simulink library "lib_transmission2"  (Simulink 4.1.1)
values from neighbouring files (symbols this model uses):
  logFlag = 1    [advSACompMaskInit.m]    (also in advSACompMaskInitR13.m)
undefined symbols (not defined in the file or in its folder): cyc_mph, fc_map_spd, fc_max_trq, fc_spd_scale, fc_trq_scale, fd_inertia, fd_loss, fd_ratio, gb_dnshift_load, gb_dnshift_spd, gb_gear_number_lookup, gb_gears_num, gb_inertia, gb_loss_const, gb_loss_input_spd_coeff, gb_loss_input_trq_coeff, gb_loss_output_spd_coeff, gb_loss_output_trq_coeff, gb_map_spd_out, gb_map_trq_in, gb_map_trq_out, gb_num_init, gb_ratio, gb_shift_delay, gb_spd_scale, gb_trq_scale, gb_upshift_load, gb_upshift_spd, htc_inertia, htc_k_adv, htc_k_adv_coast, htc_lockup, htc_lockup_load, htc_lockup_spd, htc_lu_gear_range, htc_max_coast_tr, htc_min_coast_tr, htc_pump_loss_spd, htc_pump_loss_trq_lockup, htc_pump_loss_trq_unlock, htc_sr, htc_sr_coast, htc_tr, htc_tr_coast, htc_unlock_spd, mc_map_spd, mc_max_trq, mc_overtrq_factor, mc_spd_scale, mc_trq_scale, tc_loss, tc_mc_to_fc_ratio, tx_eff_map, tx_map_spd, tx_map_trq, tx_pg_r, tx_pg_s, tx_speed_dep, vc_clutch_bool, vc_idle_spd ... (+2)
libraries: lib_controls x1, lib_etc x1, lib_controls2 x1, lib_transmission x1
(part 14 of 17)

== system lib_transmission2/gearbox <gb> old/gearbox model & interface/gearbox model/gearing (Nm) (rad/s) ==
  "output shaft torque and speed  (Nm), (rad/s)" : Inport  Port=1  LatchInput=off
  gear ratio : Inport  Port=2  LatchInput=off
  Demux : Demux  Outputs=2  BusSelectionMode=off
  Fcn1 : Fcn  Expr=1/u
  Product2 : Product  Inputs=2  Multiplication=Element-wise(.*)  SaturateOnIntegerOverflow=on
  Product3 : Product  Inputs=2  Multiplication=Element-wise(.*)  SaturateOnIntegerOverflow=on
  input shaft torque (Nm) : Outport  Port=1  InitialOutput=0
  input shaft speed (rad/s) : Outport  Port=2  InitialOutput=0
  wires:
  Product3/1 -> input shaft speed (rad/s)/1
  Product2/1 -> input shaft torque (Nm)/1
  Fcn1/1 -> Product2/2
  "output shaft torque and speed  (Nm), (rad/s)"/1 -> Demux/1
  gear ratio/1 -> Fcn1/1, Product3/2
  Demux/1 -> Product2/1
  Demux/2 -> Product3/1

== system lib_transmission2/gearbox <gb> old/gearbox model & interface/gearbox model/gearing (Nm) (rad/s)1 ==
  input shaft torque (Nm) : Inport  Port=1  LatchInput=off
  input shaft speed (rad/s) : Inport  Port=2  LatchInput=off
  gear ratio : Inport  Port=3  LatchInput=off
  Fcn1 : Fcn  Expr=1/u
  Product2 : Product  Inputs=2  Multiplication=Element-wise(.*)  SaturateOnIntegerOverflow=on
  Product3 : Product  Inputs=2  Multiplication=Element-wise(.*)  SaturateOnIntegerOverflow=on
  output shaft torque (Nm) : Outport  Port=1  InitialOutput=0
  output shaft speed (rad/s) : Outport  Port=2  InitialOutput=0
  wires:
  Fcn1/1 -> Product3/1
  gear ratio/1 -> Product2/2, Fcn1/1
  Product3/1 -> output shaft speed (rad/s)/1
  Product2/1 -> output shaft torque (Nm)/1
  input shaft torque (Nm)/1 -> Product2/1
  input shaft speed (rad/s)/1 -> Product3/2

== system lib_transmission2/gearbox <gb> old/gearbox model & interface/gearbox model/help ==

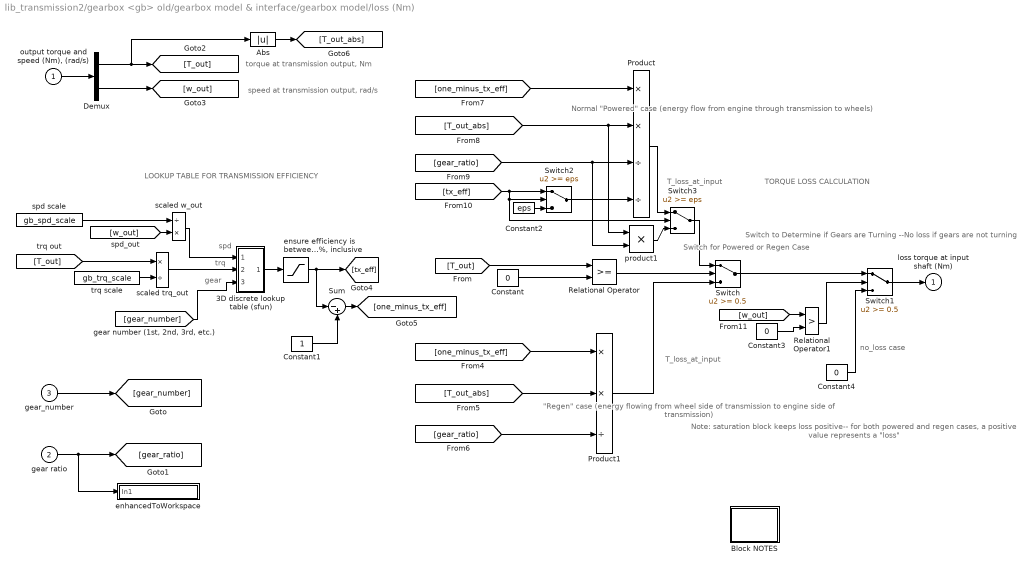
== system lib_transmission2/gearbox <gb> old/gearbox model & interface/gearbox model/loss (Nm) ==
  note: TORQUE LOSS CALCULATION
  note: gear
  note: trq
  note: spd
  note: torque at transmission output, Nm
  note: speed at transmission output, rad/s
  note: no_loss case
  note: Note: saturation block keeps
      | loss positive-- for both powered
      | and regen cases, a
      | positive value represents a "loss"
  note: Switch for Powered
      |  or Regen Case
  note: Switch to Determine
      | if Gears are Turning
      | --No loss if gears
      | are not turning
  note: Normal "Powered" case
      | (energy flow from engine
      | through transmission to wheels)
  note: T_loss_at_input
  note: "Regen" case
      | (energy flowing from
      | wheel side of transmission
      | to engine side of transmission)
  note: T_loss_at_input
  note: LOOKUP TABLE FOR TRANSMISSION EFFICIENCY
  "output torque and speed (Nm), (rad/s)" : Inport  Port=1  LatchInput=off
  gear ratio : Inport  Port=2  LatchInput=off
  gear_number : Inport  Port=3  LatchInput=off
  3D discrete lookup table (sfun) : Subsystem  mask{tx_map_spd=tx_map_spd, tx_map_trq=tx_map_trq, tx_eff_map=tx_eff_map}
      mask prompts: tx_map_spd "Row Lookup"; tx_map_trq "Column Lookup"; tx_eff_map "Lookup Matrix"
      settings: RTWFcnNameOpts=Auto  RTWFileNameOpts=Auto
  Abs : Abs  SaturateOnIntegerOverflow=on
  Block NOTES : Subsystem
      settings: RTWFcnNameOpts=Auto  RTWFileNameOpts=Auto
      mask Display: disp('Block\nNOTES')
  Constant : Constant  Value=0
  Constant1 : Constant  Value=1
  Constant2 : Constant  Value=eps
  Constant3 : Constant  Value=0
  Constant4 : Constant  Value=0
  Demux : Demux  Outputs=2  BusSelectionMode=off
  Product : Product  Inputs=**//  Multiplication=Element-wise(.*)  SaturateOnIntegerOverflow=on
  Product1 : Product  Inputs=**/  Multiplication=Element-wise(.*)  SaturateOnIntegerOverflow=on
  Relational Operator : RelationalOperator  Operator=>=
  Relational Operator1 : RelationalOperator  Operator=>
  Sum : Sum  Inputs=|-+  SaturateOnIntegerOverflow=on
  Switch : Switch  Threshold=0.5
  Switch1 : Switch  Threshold=0.5
  Switch2 : Switch  Threshold=eps
  Switch3 : Switch  Threshold=eps
  enhancedToWorkspace : Subsystem  TreatAsAtomicUnit=on  mask(enhancedToWorkspace){generalName=generalName, specificName=current_gear_ratio, logFlag=logFlag}
      mask prompts: generalName "General Name [char-evaluated]"; specificName "Specific Name [char-literal]"; logFlag "Enable flag (1=on,0=off)"
      mask help: A wrapper for the Simulink "To Workspace" block that allows you to evaluate the name of the variable to log to workspace. This is useful to avoid the double logging errors that occur when you pull in two library models that attempt to log to the same variable.
      mask init:
      | enhancedToWsMaker
      settings: CopyFcn=breakLinkCopyFcn  ParentCloseFcn=breakLinkParCloseFcn  RTWFcnNameOpts=Auto  RTWFileNameOpts=Auto
      mask Help:
      | <h2>Enhanced To Workspace Block</h2>
      | <h3>Parameters</h3>
      | <UL>
      | <li><b>General Name:</b> This is the more general name of the variable. Variables are saved to the workspace as <i>generalName_specificName</i>. Note that this is an evaluated variable. If you would like to type in the value directly, it must be surrounded with single quotes. Otherwise you can input the name of a variable containing a char string.</li>
      | <li><b>Specific Name:</b> This is the specific name of the variable. Note that this is input as a char literal (i.e., you don't need quotes).</li>
      | <li><b>Enable Flag:</b> This flag should have the value of 0 or 1. If 0, the variable will not be logged to the workspace. If 1, the variable will be logged. This is done so that variable logging can be turned off to improve speed.</li>
      | </ul>
      | <h3>Overview</h3>
      | <p>The enhanced to workspace block was put together to allow one to dynamically resolve variable names at run time in simulink. This is most powerful when used in conjunction with a masked subsystem to allow multiple instances of that masked subsytem to be used in the same model. The strategy is to set the generalName in the block mask which will allow the block to change the general name for all variable logging on the fly.
      | <h3>Helper Files</h3>
      | <p>Three m-files are required by the enhancedToWorkspace block. These files are located in the &lt; ADVISOR root &gt;/GUI directory :
      | <ul>
      | <li><i>enhancedToWsMaker.m</i> This file runs the mask initialization for the block</li>
      | <li><i>breakLinkCopyFcn.m</i> This file is used by the block callback when the simulink block is copied. It is necessary to break the link to the enhancedToWorkspace similar to the To Workspace block in order for it to be able to configure itself. (Try copying simulink's To Workspace block--it is impossible to make a link)</li>
      | <li><i>breakLinkParCloseFcn.m</i> This file is similar to the breakLinkCopyFcn and is used when a parent system is closed</li>
      | </ul>
      | <hr>
      | 
      | <p>Created 2003-Jan-21, Michael Patrick O'Keefe, NREL</p>
      | 
      | <!--
      | <VARDEF>
      | <H3>var_name</H3>
      | <UL>
      | <LI><B>data type</B> data type here</LI>
      | <LI><B>units</B> units here</LI>
      | <LI><B>vehicle type</B> vehicle type here</LI>
      | <LI><B>description</B> description here</LI>
      | </UL>
      | </VARDEF>
      | -->
      mask Display: disp([generalName,'_',specificName])
  "ensure efficiency is between  0% and 100%, inclusive" : Saturate  UpperLimit=1  LowerLimit=0  LinearizeAsGain=on
  product1 : Product  Inputs=2  Multiplication=Element-wise(.*)  SaturateOnIntegerOverflow=on
  scaled trq_out : Product  Inputs=*/  Multiplication=Element-wise(.*)  SaturateOnIntegerOverflow=on
  scaled w_out : Product  Inputs=/*  Multiplication=Element-wise(.*)  SaturateOnIntegerOverflow=on
  spd scale : Constant  Value=gb_spd_scale
  trq scale : Constant  Value=gb_trq_scale
  loss torque at input shaft (Nm) : Outport  Port=1  InitialOutput=0
  wires:
  product1/1 -> Switch3/3
  Product/1 -> Switch3/1
  Switch3/1 -> Switch/1
  Constant2/1 -> Switch2/3
  [tx_eff] -> Switch3/2, Switch2/2, Switch2/1
  Switch2/1 -> Product/4
  gear_number/1 -> [gear_number]
  gear ratio/1 -> [gear_ratio], enhancedToWorkspace/1(In1)
  spd scale/1 -> scaled w_out/1
  [w_out] -> scaled w_out/2
  Sum/1 -> [one_minus_tx_eff]
  Constant1/1 -> Sum/2
  trq scale/1 -> scaled trq_out/2
  scaled trq_out/1 -> 3D discrete lookup table (sfun)/2(lookup trq (Nm))
  [T_out] -> scaled trq_out/1
  scaled w_out/1 -> 3D discrete lookup table (sfun)/1(lookup speed (rad/s))
  "ensure efficiency is between  0% and 100%, inclusive"/1 -> Sum/1, [tx_eff]
  3D discrete lookup table (sfun)/1(tx_eff) -> "ensure efficiency is between  0% and 100%, inclusive"/1
  Switch/1 -> Switch1/1
  Abs/1 -> [T_out_abs]
  Demux/1 -> Abs/1, [T_out]
  Relational Operator1/1 -> Switch1/2
  Constant3/1 -> Relational Operator1/2
  [w_out] -> Relational Operator1/1
  Constant4/1 -> Switch1/3
  Switch1/1 -> loss torque at input shaft (Nm)/1
  [gear_ratio] -> product1/2, Product/3
  [T_out_abs] -> product1/1, Product/2
  [one_minus_tx_eff] -> Product/1
  [T_out_abs] -> Product1/2
  [gear_ratio] -> Product1/3
  [one_minus_tx_eff] -> Product1/1
  Product1/1 -> Switch/3
  [T_out] -> Relational Operator/1
  Constant/1 -> Relational Operator/2
  Relational Operator/1 -> Switch/2
  [gear_number] -> 3D discrete lookup table (sfun)/3("gear_number  (e.g., 1, 2, 3)")
  Demux/2 -> [w_out]
  "output torque and speed (Nm), (rad/s)"/1 -> Demux/1

== system lib_transmission2/hydraulic torque converter <htc>/conventional HTC  and Interface/htc model/SR ==
  T,w req out : Inport  Port=1  LatchInput=off
  w in : Inport  Port=2  LatchInput=off
  >0 : Saturate  UpperLimit=inf  LowerLimit=eps  LinearizeAsGain=on
  Constant : Constant  Orientation=left  Value=0
  Constant1 : Constant  Value=vc_idle_spd+eps
  Constant3 : Constant  Value=1
  K_adv : Subsystem
      settings: RTWFcnNameOpts=Auto  RTWFileNameOpts=Auto
  K_adv_coast : Subsystem
      settings: RTWFcnNameOpts=Auto  RTWFileNameOpts=Auto
  Logical Operator : Logic  Operator=NOT  Inputs=1
  Logical Operator1 : Logic  Operator=NOT  Inputs=1
  MinMax : MinMax  Function=min  Inputs=2
  Relational Operator : RelationalOperator  Operator=>=
  SR Look-Up Table SR=wout/win : Lookup  InputValues=htc_k_adv  OutputValues=htc_sr
  SR Look-Up Table SR=wout/win coast : Lookup  InputValues=fliplr(htc_k_adv_coast)  OutputValues=fliplr(htc_sr_coast)
  SRmax= wout/win,min : Product  Inputs=*/  Multiplication=Element-wise(.*)  SaturateOnIntegerOverflow=on
  T : Selector  InputType=Vector  ElementSrc=Internal  Elements=1  RowSrc=Internal  Rows=1  ColumnSrc=Internal  Columns=1  InputPortWidth=2
  enhancedToWorkspace1 : Subsystem  TreatAsAtomicUnit=on  mask(enhancedToWorkspace){generalName=generalName, specificName=coasting, logFlag=logFlag}
      mask prompts: generalName "General Name [char-evaluated]"; specificName "Specific Name [char-literal]"; logFlag "Enable flag (1=on,0=off)"
      mask help: A wrapper for the Simulink "To Workspace" block that allows you to evaluate the name of the variable to log to workspace. This is useful to avoid the double logging errors that occur when you pull in two library models that attempt to log to the same variable.
      mask init:
      | enhancedToWsMaker
      settings: CopyFcn=breakLinkCopyFcn  ParentCloseFcn=breakLinkParCloseFcn  RTWFcnNameOpts=Auto  RTWFileNameOpts=Auto
      mask Help:
      | <h2>Enhanced To Workspace Block</h2>
      | <h3>Parameters</h3>
      | <UL>
      | <li><b>General Name:</b> This is the more general name of the variable. Variables are saved to the workspace as <i>generalName_specificName</i>. Note that this is an evaluated variable. If you would like to type in the value directly, it must be surrounded with single quotes. Otherwise you can input the name of a variable containing a char string.</li>
      | <li><b>Specific Name:</b> This is the specific name of the variable. Note that this is input as a char literal (i.e., you don't need quotes).</li>
      | <li><b>Enable Flag:</b> This flag should have the value of 0 or 1. If 0, the variable will not be logged to the workspace. If 1, the variable will be logged. This is done so that variable logging can be turned off to improve speed.</li>
      | </ul>
      | <h3>Overview</h3>
      | <p>The enhanced to workspace block was put together to allow one to dynamically resolve variable names at run time in simulink. This is most powerful when used in conjunction with a masked subsystem to allow multiple instances of that masked subsytem to be used in the same model. The strategy is to set the generalName in the block mask which will allow the block to change the general name for all variable logging on the fly.
      | <h3>Helper Files</h3>
      | <p>Three m-files are required by the enhancedToWorkspace block. These files are located in the &lt; ADVISOR root &gt;/GUI directory :
      | <ul>
      | <li><i>enhancedToWsMaker.m</i> This file runs the mask initialization for the block</li>
      | <li><i>breakLinkCopyFcn.m</i> This file is used by the block callback when the simulink block is copied. It is necessary to break the link to the enhancedToWorkspace similar to the To Workspace block in order for it to be able to configure itself. (Try copying simulink's To Workspace block--it is impossible to make a link)</li>
      | <li><i>breakLinkParCloseFcn.m</i> This file is similar to the breakLinkCopyFcn and is used when a parent system is closed</li>
      | </ul>
      | <hr>
      | 
      | <p>Created 2003-Jan-21, Michael Patrick O'Keefe, NREL</p>
      | 
      | <!--
      | <VARDEF>
      | <H3>var_name</H3>
      | <UL>
      | <LI><B>data type</B> data type here</LI>
      | <LI><B>units</B> units here</LI>
      | <LI><B>vehicle type</B> vehicle type here</LI>
      | <LI><B>description</B> description here</LI>
      | </UL>
      | </VARDEF>
      | -->
      mask Display: disp([generalName,'_',specificName])
  enhancedToWorkspace2 : Subsystem  TreatAsAtomicUnit=on  mask(enhancedToWorkspace){generalName=generalName, specificName=locked, logFlag=logFlag}
      mask prompts: generalName "General Name [char-evaluated]"; specificName "Specific Name [char-literal]"; logFlag "Enable flag (1=on,0=off)"
      mask help: A wrapper for the Simulink "To Workspace" block that allows you to evaluate the name of the variable to log to workspace. This is useful to avoid the double logging errors that occur when you pull in two library models that attempt to log to the same variable.
      mask init:
      | enhancedToWsMaker
      settings: CopyFcn=breakLinkCopyFcn  ParentCloseFcn=breakLinkParCloseFcn  RTWFcnNameOpts=Auto  RTWFileNameOpts=Auto
      mask Help:
      | <h2>Enhanced To Workspace Block</h2>
      | <h3>Parameters</h3>
      | <UL>
      | <li><b>General Name:</b> This is the more general name of the variable. Variables are saved to the workspace as <i>generalName_specificName</i>. Note that this is an evaluated variable. If you would like to type in the value directly, it must be surrounded with single quotes. Otherwise you can input the name of a variable containing a char string.</li>
      | <li><b>Specific Name:</b> This is the specific name of the variable. Note that this is input as a char literal (i.e., you don't need quotes).</li>
      | <li><b>Enable Flag:</b> This flag should have the value of 0 or 1. If 0, the variable will not be logged to the workspace. If 1, the variable will be logged. This is done so that variable logging can be turned off to improve speed.</li>
      | </ul>
      | <h3>Overview</h3>
      | <p>The enhanced to workspace block was put together to allow one to dynamically resolve variable names at run time in simulink. This is most powerful when used in conjunction with a masked subsystem to allow multiple instances of that masked subsytem to be used in the same model. The strategy is to set the generalName in the block mask which will allow the block to change the general name for all variable logging on the fly.
      | <h3>Helper Files</h3>
      | <p>Three m-files are required by the enhancedToWorkspace block. These files are located in the &lt; ADVISOR root &gt;/GUI directory :
      | <ul>
      | <li><i>enhancedToWsMaker.m</i> This file runs the mask initialization for the block</li>
      | <li><i>breakLinkCopyFcn.m</i> This file is used by the block callback when the simulink block is copied. It is necessary to break the link to the enhancedToWorkspace similar to the To Workspace block in order for it to be able to configure itself. (Try copying simulink's To Workspace block--it is impossible to make a link)</li>
      | <li><i>breakLinkParCloseFcn.m</i> This file is similar to the breakLinkCopyFcn and is used when a parent system is closed</li>
      | </ul>
      | <hr>
      | 
      | <p>Created 2003-Jan-21, Michael Patrick O'Keefe, NREL</p>
      | 
      | <!--
      | <VARDEF>
      | <H3>var_name</H3>
      | <UL>
      | <LI><B>data type</B> data type here</LI>
      | <LI><B>units</B> units here</LI>
      | <LI><B>vehicle type</B> vehicle type here</LI>
      | <LI><B>description</B> description here</LI>
      | </UL>
      | </VARDEF>
      | -->
      mask Display: disp([generalName,'_',specificName])
  if coasting : Switch  Threshold=eps
  "locked up, then SR=1" : Switch  Threshold=eps
  min,max : Saturate  UpperLimit=inf  LowerLimit=1  LinearizeAsGain=on
  shifting SR : Subsystem
      settings: RTWFcnNameOpts=Auto  RTWFileNameOpts=Auto
  wout,req : Selector  InputType=Vector  ElementSrc=Internal  Elements=2  RowSrc=Internal  Rows=1  ColumnSrc=Internal  Columns=1  InputPortWidth=2
  SR : Outport  Port=1  InitialOutput=0
  coasting : Outport  Port=2  InitialOutput=0
  wires:
  K_adv/1(K_adv) -> SR Look-Up Table SR=wout/win/1
  Logical Operator1/1 -> coasting/1, enhancedToWorkspace1/1(In1)
  >0/1 -> SR/1
  if coasting/1 -> >0/1
  K_adv_coast/1(K_adv_coast) -> SR Look-Up Table SR=wout/win coast/1
  MinMax/1 -> if coasting/3
  min,max/1 -> MinMax/1
  wout,req/1 -> SRmax= wout/win,min/1
  Constant1/1 -> SRmax= wout/win,min/2
  SRmax= wout/win,min/1 -> MinMax/2
  shifting SR/1(SR limited) -> if coasting/1
  "locked up, then SR=1"/1 -> shifting SR/3(SR)
  w in/1 -> shifting SR/2(w in)
  SR Look-Up Table SR=wout/win/1 -> "locked up, then SR=1"/1
  Constant3/1 -> "locked up, then SR=1"/3
  Logical Operator/1 -> "locked up, then SR=1"/2
  Relational Operator/1 -> Logical Operator1/1, if coasting/2
  T/1 -> Relational Operator/1
  Constant/1 -> Relational Operator/2
  SR Look-Up Table SR=wout/win coast/1 -> min,max/1
  T,w req out/1 -> shifting SR/1(T,w req out), K_adv/1("Req'd output trq and spd (Nm), (rad/s)"), wout,req/1, K_adv_coast/1("Req'd output trq and spd (Nm), (rad/s)"), T/1
  [locked_up] -> Logical Operator/1, enhancedToWorkspace2/1(In1)

== system lib_transmission2/hydraulic torque converter <htc>/conventional HTC  and Interface/htc model/T, shifting ==
  TR : Inport  Port=1  LatchInput=off
  Req'd  input trq : Inport  Port=2  LatchInput=off
  Req'd output trq : Inport  Port=3  LatchInput=off
  htc_spd_in_a : Inport  Port=4  LatchInput=off
  SR : Inport  Port=5  LatchInput=off
  Memory : Memory  X0=0  InheritSampleTime=off
      settings: RTWStateStorageClass=Auto
  Memory1 : Memory  X0=0  InheritSampleTime=off
      settings: RTWStateStorageClass=Auto
  MinMax : MinMax  Function=min  Inputs=2
  TR Look-Up Table TR=Tout/Tin : Lookup  InputValues=htc_sr  OutputValues=htc_tr
  T_max : Subsystem
      settings: RTWFcnNameOpts=Auto  RTWFileNameOpts=Auto
  Tin*TR= Tout,req : Product  Inputs=2  Multiplication=Element-wise(.*)  SaturateOnIntegerOverflow=on
  engine speed estimator : Subsystem
      settings: RTWFcnNameOpts=Auto  RTWFileNameOpts=Auto
  "shifting, override zero Trequest" : Switch  Threshold=eps
  T req : Outport  Port=1
  wires:
  Tin*TR= Tout,req/1 -> Memory/1
  TR/1 -> Tin*TR= Tout,req/2
  Req'd  input trq/1 -> Tin*TR= Tout,req/1
  Memory/1 -> "shifting, override zero Trequest"/1
  T_max/1(T_max max gain from htc) -> MinMax/2
  "shifting, override zero Trequest"/1 -> MinMax/1
  TR Look-Up Table TR=Tout/Tin/1 -> T_max/2(TR)
  MinMax/1 -> T req/1
  engine speed estimator/1(Out1) -> T_max/1(w_APU)
  Memory1/1 -> TR Look-Up Table TR=Tout/Tin/1
  SR/1 -> Memory1/1
  htc_spd_in_a/1 -> engine speed estimator/1(htc_spd_in_a)
  Req'd output trq/1 -> "shifting, override zero Trequest"/3
  [shifting] -> "shifting, override zero Trequest"/2

== system lib_transmission2/hydraulic torque converter <htc>/conventional HTC  and Interface/htc model/TR ==
  SR : Inport  Port=1  LatchInput=off
  coasting : Inport  Port=2  LatchInput=off
  1/SR*TR  for coast : Fcn  Expr=1/u
  Constant3 : Constant  Value=1
  Logical Operator : Logic  Operator=NOT  Inputs=1
  Logical Operator1 : Logic  Operator=NOT  Inputs=1
  TR Look-Up Table TR=Tout/Tin : Lookup  InputValues=htc_sr  OutputValues=htc_tr
  TR Look-Up Table TR=Tout/Tin coast : Lookup  InputValues=htc_sr_coast  OutputValues=htc_tr_coast
  effic=SR*TR : Product  Inputs=**  Multiplication=Element-wise(.*)  SaturateOnIntegerOverflow=on
  enhancedToWorkspace2 : Subsystem  TreatAsAtomicUnit=on  mask(enhancedToWorkspace){generalName=generalName, specificName=efficiency, logFlag=logFlag}
      mask prompts: generalName "General Name [char-evaluated]"; specificName "Specific Name [char-literal]"; logFlag "Enable flag (1=on,0=off)"
      mask help: A wrapper for the Simulink "To Workspace" block that allows you to evaluate the name of the variable to log to workspace. This is useful to avoid the double logging errors that occur when you pull in two library models that attempt to log to the same variable.
      mask init:
      | enhancedToWsMaker
      settings: CopyFcn=breakLinkCopyFcn  ParentCloseFcn=breakLinkParCloseFcn  RTWFcnNameOpts=Auto  RTWFileNameOpts=Auto
      mask Help:
      | <h2>Enhanced To Workspace Block</h2>
      | <h3>Parameters</h3>
      | <UL>
      | <li><b>General Name:</b> This is the more general name of the variable. Variables are saved to the workspace as <i>generalName_specificName</i>. Note that this is an evaluated variable. If you would like to type in the value directly, it must be surrounded with single quotes. Otherwise you can input the name of a variable containing a char string.</li>
      | <li><b>Specific Name:</b> This is the specific name of the variable. Note that this is input as a char literal (i.e., you don't need quotes).</li>
      | <li><b>Enable Flag:</b> This flag should have the value of 0 or 1. If 0, the variable will not be logged to the workspace. If 1, the variable will be logged. This is done so that variable logging can be turned off to improve speed.</li>
      | </ul>
      | <h3>Overview</h3>
      | <p>The enhanced to workspace block was put together to allow one to dynamically resolve variable names at run time in simulink. This is most powerful when used in conjunction with a masked subsystem to allow multiple instances of that masked subsytem to be used in the same model. The strategy is to set the generalName in the block mask which will allow the block to change the general name for all variable logging on the fly.
      | <h3>Helper Files</h3>
      | <p>Three m-files are required by the enhancedToWorkspace block. These files are located in the &lt; ADVISOR root &gt;/GUI directory :
      | <ul>
      | <li><i>enhancedToWsMaker.m</i> This file runs the mask initialization for the block</li>
      | <li><i>breakLinkCopyFcn.m</i> This file is used by the block callback when the simulink block is copied. It is necessary to break the link to the enhancedToWorkspace similar to the To Workspace block in order for it to be able to configure itself. (Try copying simulink's To Workspace block--it is impossible to make a link)</li>
      | <li><i>breakLinkParCloseFcn.m</i> This file is similar to the breakLinkCopyFcn and is used when a parent system is closed</li>
      | </ul>
      | <hr>
      | 
      | <p>Created 2003-Jan-21, Michael Patrick O'Keefe, NREL</p>
      | 
      | <!--
      | <VARDEF>
      | <H3>var_name</H3>
      | <UL>
      | <LI><B>data type</B> data type here</LI>
      | <LI><B>units</B> units here</LI>
      | <LI><B>vehicle type</B> vehicle type here</LI>
      | <LI><B>description</B> description here</LI>
      | </UL>
      | </VARDEF>
      | -->
      mask Display: disp([generalName,'_',specificName])
  if coasting : Switch  Threshold=eps
  if coasting1 : Switch  Threshold=eps
  "locked up, then TR=1" : Switch  Threshold=eps
  min,max : Saturate  UpperLimit=htc_max_coast_tr  LowerLimit=htc_min_coast_tr  LinearizeAsGain=on
  TR : Outport  Port=1  InitialOutput=0
  tag scope: htc_efficiency=scoped
  wires:
  if coasting1/1 -> [htc_efficiency], enhancedToWorkspace2/1(In1)
  1/SR*TR  for coast/1 -> if coasting1/3
  effic=SR*TR/1 -> 1/SR*TR  for coast/1, if coasting1/1
  Logical Operator1/1 -> if coasting1/2, if coasting/2
  if coasting/1 -> effic=SR*TR/2, TR/1
  coasting/1 -> Logical Operator1/1
  SR/1 -> effic=SR*TR/1, TR Look-Up Table TR=Tout/Tin/1, TR Look-Up Table TR=Tout/Tin coast/1
  min,max/1 -> if coasting/3
  TR Look-Up Table TR=Tout/Tin coast/1 -> min,max/1
  "locked up, then TR=1"/1 -> if coasting/1
  Logical Operator/1 -> "locked up, then TR=1"/2
  [locked_up] -> Logical Operator/1
  Constant3/1 -> "locked up, then TR=1"/3
  TR Look-Up Table TR=Tout/Tin/1 -> "locked up, then TR=1"/1

== system lib_transmission2/hydraulic torque converter <htc>/conventional HTC  and Interface/htc model/effect of inertia (Nm) ==
  note: This block computes the torque required to overcome the inertia of the
      | turbine (plus 1/2 fluid in htc).
  turbine/output speed (rad/s) : Inport  Port=1  LatchInput=off
  Constant : Constant  Value=htc_inertia
  Product : Product  Inputs=2  Multiplication=Element-wise(.*)  SaturateOnIntegerOverflow=on
  d/dt : Derivative
  inertia torque (Nm) : Outport  Port=1  InitialOutput=0
  wires:
  Product/1 -> inertia torque (Nm)/1
  Constant/1 -> Product/2
  turbine/output speed (rad/s)/1 -> d/dt/1
  d/dt/1 -> Product/1

== system lib_transmission2/hydraulic torque converter <htc>/conventional HTC  and Interface/htc model/enhancedToWorkspace ==
  In1 : Inport  Port=1  LatchInput=off
  To Workspace : ToWorkspace  VariableName=htc_trq_in_a  SampleTime=-1  SaveFormat=Array
  wires:
  In1/1 -> To Workspace/1

== system lib_transmission2/hydraulic torque converter <htc>/conventional HTC  and Interface/htc model/enhancedToWorkspace1 ==
  In1 : Inport  Port=1  LatchInput=off
  To Workspace : ToWorkspace  VariableName=htc_spd_in_a  SampleTime=-1  SaveFormat=Array
  wires:
  In1/1 -> To Workspace/1

== system lib_transmission2/hydraulic torque converter <htc>/conventional HTC  and Interface/htc model/enhancedToWorkspace10 ==
  In1 : Inport  Port=1  LatchInput=off
  To Workspace : ToWorkspace  VariableName=htc_spd_out_a  SampleTime=-1  SaveFormat=Array
  wires:
  In1/1 -> To Workspace/1

== system lib_transmission2/hydraulic torque converter <htc>/conventional HTC  and Interface/htc model/enhancedToWorkspace2 ==
  In1 : Inport  Port=1  LatchInput=off
  To Workspace : ToWorkspace  VariableName=htc_trq_out_r  SampleTime=-1  SaveFormat=Array
  wires:
  In1/1 -> To Workspace/1

== system lib_transmission2/hydraulic torque converter <htc>/conventional HTC  and Interface/htc model/enhancedToWorkspace3 ==
  In1 : Inport  Port=1  LatchInput=off
  To Workspace : ToWorkspace  VariableName=htc_spd_out_r  SampleTime=-1  SaveFormat=Array
  wires:
  In1/1 -> To Workspace/1

== system lib_transmission2/hydraulic torque converter <htc>/conventional HTC  and Interface/htc model/enhancedToWorkspace4 ==
  In1 : Inport  Port=1  LatchInput=off
  To Workspace : ToWorkspace  VariableName=htc_sr_hist  SampleTime=-1  SaveFormat=Array
  wires:
  In1/1 -> To Workspace/1

== system lib_transmission2/hydraulic torque converter <htc>/conventional HTC  and Interface/htc model/enhancedToWorkspace5 ==
  In1 : Inport  Port=1  LatchInput=off
  To Workspace : ToWorkspace  VariableName=htc_tr_hist  SampleTime=-1  SaveFormat=Array
  wires:
  In1/1 -> To Workspace/1

== system lib_transmission2/hydraulic torque converter <htc>/conventional HTC  and Interface/htc model/enhancedToWorkspace6 ==
  In1 : Inport  Port=1  LatchInput=off
  To Workspace : ToWorkspace  VariableName=htc_spd_in_r  SampleTime=-1  SaveFormat=Array
  wires:
  In1/1 -> To Workspace/1

== system lib_transmission2/hydraulic torque converter <htc>/conventional HTC  and Interface/htc model/enhancedToWorkspace7 ==
  In1 : Inport  Port=1  LatchInput=off
  To Workspace : ToWorkspace  VariableName=htc_trq_in_r  SampleTime=-1  SaveFormat=Array
  wires:
  In1/1 -> To Workspace/1

== system lib_transmission2/hydraulic torque converter <htc>/conventional HTC  and Interface/htc model/enhancedToWorkspace8 ==
  In1 : Inport  Port=1  LatchInput=off
  To Workspace : ToWorkspace  VariableName=htc_trq_inertia  SampleTime=-1  SaveFormat=Array
  wires:
  In1/1 -> To Workspace/1

== system lib_transmission2/hydraulic torque converter <htc>/conventional HTC  and Interface/htc model/enhancedToWorkspace9 ==
  In1 : Inport  Port=1  LatchInput=off
  To Workspace : ToWorkspace  VariableName=htc_trq_out_a  SampleTime=-1  SaveFormat=Array
  wires:
  In1/1 -> To Workspace/1

== system lib_transmission2/hydraulic torque converter <htc> HEV/HTC for parallel HEV and Interface/model for parallel HEV/Block NOTES ==
  note: This block predicts the relative speed of the HTC input (pump) and output
      | (turbine).  Torque converter lockup is modeled.

== system lib_transmission2/hydraulic torque converter <htc> HEV/HTC for parallel HEV and Interface/model for parallel HEV/SR ==
  T,w req out : Inport  Port=1  LatchInput=off
  w in : Inport  Port=2  LatchInput=off
  >0 : Saturate  UpperLimit=inf  LowerLimit=eps  LinearizeAsGain=on
  Constant : Constant  Orientation=left  Value=0
  Constant1 : Constant  Value=vc_idle_spd+eps
  Constant3 : Constant  Value=1
  K_adv : Subsystem
      settings: RTWFcnNameOpts=Auto  RTWFileNameOpts=Auto
  K_adv_coast : Subsystem
      settings: RTWFcnNameOpts=Auto  RTWFileNameOpts=Auto
  Logical Operator : Logic  Operator=NOT  Inputs=1
  Logical Operator1 : Logic  Operator=NOT  Inputs=1
  MinMax : MinMax  Function=min  Inputs=2
  Relational Operator : RelationalOperator  Operator=>=
  SR Look-Up Table SR=wout/win : Lookup  InputValues=htc_k_adv  OutputValues=htc_sr
  SR Look-Up Table SR=wout/win coast : Lookup  InputValues=fliplr(htc_k_adv_coast)  OutputValues=fliplr(htc_sr_coast)
  SRmax= wout/win,min : Product  Inputs=*/  Multiplication=Element-wise(.*)  SaturateOnIntegerOverflow=on
  T : Selector  InputType=Vector  ElementSrc=Internal  Elements=1  RowSrc=Internal  Rows=1  ColumnSrc=Internal  Columns=1  InputPortWidth=2
  enhancedToWorkspace : Subsystem  TreatAsAtomicUnit=on  mask(enhancedToWorkspace){generalName=generalName, specificName=locked, logFlag=logFlag}
      mask prompts: generalName "General Name [char-evaluated]"; specificName "Specific Name [char-literal]"; logFlag "Enable flag (1=on,0=off)"
      mask help: A wrapper for the Simulink "To Workspace" block that allows you to evaluate the name of the variable to log to workspace. This is useful to avoid the double logging errors that occur when you pull in two library models that attempt to log to the same variable.
      mask init:
      | enhancedToWsMaker
      settings: CopyFcn=breakLinkCopyFcn  ParentCloseFcn=breakLinkParCloseFcn  RTWFcnNameOpts=Auto  RTWFileNameOpts=Auto
      mask Help:
      | <h2>Enhanced To Workspace Block</h2>
      | <h3>Parameters</h3>
      | <UL>
      | <li><b>General Name:</b> This is the more general name of the variable. Variables are saved to the workspace as <i>generalName_specificName</i>. Note that this is an evaluated variable. If you would like to type in the value directly, it must be surrounded with single quotes. Otherwise you can input the name of a variable containing a char string.</li>
      | <li><b>Specific Name:</b> This is the specific name of the variable. Note that this is input as a char literal (i.e., you don't need quotes).</li>
      | <li><b>Enable Flag:</b> This flag should have the value of 0 or 1. If 0, the variable will not be logged to the workspace. If 1, the variable will be logged. This is done so that variable logging can be turned off to improve speed.</li>
      | </ul>
      | <h3>Overview</h3>
      | <p>The enhanced to workspace block was put together to allow one to dynamically resolve variable names at run time in simulink. This is most powerful when used in conjunction with a masked subsystem to allow multiple instances of that masked subsytem to be used in the same model. The strategy is to set the generalName in the block mask which will allow the block to change the general name for all variable logging on the fly.
      | <h3>Helper Files</h3>
      | <p>Three m-files are required by the enhancedToWorkspace block. These files are located in the &lt; ADVISOR root &gt;/GUI directory :
      | <ul>
      | <li><i>enhancedToWsMaker.m</i> This file runs the mask initialization for the block</li>
      | <li><i>breakLinkCopyFcn.m</i> This file is used by the block callback when the simulink block is copied. It is necessary to break the link to the enhancedToWorkspace similar to the To Workspace block in order for it to be able to configure itself. (Try copying simulink's To Workspace block--it is impossible to make a link)</li>
      | <li><i>breakLinkParCloseFcn.m</i> This file is similar to the breakLinkCopyFcn and is used when a parent system is closed</li>
      | </ul>
      | <hr>
      | 
      | <p>Created 2003-Jan-21, Michael Patrick O'Keefe, NREL</p>
      | 
      | <!--
      | <VARDEF>
      | <H3>var_name</H3>
      | <UL>
      | <LI><B>data type</B> data type here</LI>
      | <LI><B>units</B> units here</LI>
      | <LI><B>vehicle type</B> vehicle type here</LI>
      | <LI><B>description</B> description here</LI>
      | </UL>
      | </VARDEF>
      | -->
      mask Display: disp([generalName,'_',specificName])
  enhancedToWorkspace1 : Subsystem  TreatAsAtomicUnit=on  mask(enhancedToWorkspace){generalName=generalName, specificName=coasting, logFlag=logFlag}
      mask prompts: generalName "General Name [char-evaluated]"; specificName "Specific Name [char-literal]"; logFlag "Enable flag (1=on,0=off)"
      mask help: A wrapper for the Simulink "To Workspace" block that allows you to evaluate the name of the variable to log to workspace. This is useful to avoid the double logging errors that occur when you pull in two library models that attempt to log to the same variable.
      mask init:
      | enhancedToWsMaker
      settings: CopyFcn=breakLinkCopyFcn  ParentCloseFcn=breakLinkParCloseFcn  RTWFcnNameOpts=Auto  RTWFileNameOpts=Auto
      mask Help:
      | <h2>Enhanced To Workspace Block</h2>
      | <h3>Parameters</h3>
      | <UL>
      | <li><b>General Name:</b> This is the more general name of the variable. Variables are saved to the workspace as <i>generalName_specificName</i>. Note that this is an evaluated variable. If you would like to type in the value directly, it must be surrounded with single quotes. Otherwise you can input the name of a variable containing a char string.</li>
      | <li><b>Specific Name:</b> This is the specific name of the variable. Note that this is input as a char literal (i.e., you don't need quotes).</li>
      | <li><b>Enable Flag:</b> This flag should have the value of 0 or 1. If 0, the variable will not be logged to the workspace. If 1, the variable will be logged. This is done so that variable logging can be turned off to improve speed.</li>
      | </ul>
      | <h3>Overview</h3>
      | <p>The enhanced to workspace block was put together to allow one to dynamically resolve variable names at run time in simulink. This is most powerful when used in conjunction with a masked subsystem to allow multiple instances of that masked subsytem to be used in the same model. The strategy is to set the generalName in the block mask which will allow the block to change the general name for all variable logging on the fly.
      | <h3>Helper Files</h3>
      | <p>Three m-files are required by the enhancedToWorkspace block. These files are located in the &lt; ADVISOR root &gt;/GUI directory :
      | <ul>
      | <li><i>enhancedToWsMaker.m</i> This file runs the mask initialization for the block</li>
      | <li><i>breakLinkCopyFcn.m</i> This file is used by the block callback when the simulink block is copied. It is necessary to break the link to the enhancedToWorkspace similar to the To Workspace block in order for it to be able to configure itself. (Try copying simulink's To Workspace block--it is impossible to make a link)</li>
      | <li><i>breakLinkParCloseFcn.m</i> This file is similar to the breakLinkCopyFcn and is used when a parent system is closed</li>
      | </ul>
      | <hr>
      | 
      | <p>Created 2003-Jan-21, Michael Patrick O'Keefe, NREL</p>
      | 
      | <!--
      | <VARDEF>
      | <H3>var_name</H3>
      | <UL>
      | <LI><B>data type</B> data type here</LI>
      | <LI><B>units</B> units here</LI>
      | <LI><B>vehicle type</B> vehicle type here</LI>
      | <LI><B>description</B> description here</LI>
      | </UL>
      | </VARDEF>
      | -->
      mask Display: disp([generalName,'_',specificName])
  if coasting : Switch  Threshold=eps
  "locked up, then SR=1" : Switch  Threshold=eps
  min,max : Saturate  UpperLimit=inf  LowerLimit=1  LinearizeAsGain=on
  shifting SR : Subsystem
      settings: RTWFcnNameOpts=Auto  RTWFileNameOpts=Auto
  wout,req : Selector  InputType=Vector  ElementSrc=Internal  Elements=2  RowSrc=Internal  Rows=1  ColumnSrc=Internal  Columns=1  InputPortWidth=2
  SR : Outport  Port=1  InitialOutput=0
  coasting : Outport  Port=2  InitialOutput=0
  wires:
  K_adv/1(K_adv) -> SR Look-Up Table SR=wout/win/1
  Logical Operator1/1 -> coasting/1, enhancedToWorkspace1/1(In1)
  >0/1 -> SR/1
  if coasting/1 -> >0/1
  K_adv_coast/1(K_adv_coast) -> SR Look-Up Table SR=wout/win coast/1
  MinMax/1 -> if coasting/3
  min,max/1 -> MinMax/1
  wout,req/1 -> SRmax= wout/win,min/1
  Constant1/1 -> SRmax= wout/win,min/2
  SRmax= wout/win,min/1 -> MinMax/2
  shifting SR/1(SR limited) -> if coasting/1
  "locked up, then SR=1"/1 -> shifting SR/3(SR)
  w in/1 -> shifting SR/2(w in)
  SR Look-Up Table SR=wout/win/1 -> "locked up, then SR=1"/1
  Constant3/1 -> "locked up, then SR=1"/3
  Logical Operator/1 -> "locked up, then SR=1"/2
  T/1 -> Relational Operator/1
  Constant/1 -> Relational Operator/2
  SR Look-Up Table SR=wout/win coast/1 -> min,max/1
  T,w req out/1 -> shifting SR/1(T,w req out), K_adv/1("Req'd output trq and spd (Nm), (rad/s)"), wout,req/1, K_adv_coast/1("Req'd output trq and spd (Nm), (rad/s)"), T/1
  [locked_up] -> Logical Operator/1, enhancedToWorkspace/1(In1)
  Relational Operator/1 -> Logical Operator1/1, if coasting/2

== system lib_transmission2/hydraulic torque converter <htc> HEV/HTC for parallel HEV and Interface/model for parallel HEV/T, shifting ==
  TR : Inport  Port=1  LatchInput=off
  Req'd  input trq : Inport  Port=2  LatchInput=off
  Req'd output trq : Inport  Port=3  LatchInput=off
  htc_spd_in_a : Inport  Port=4  LatchInput=off
  SR : Inport  Port=5  LatchInput=off
  Memory : Memory  X0=0  InheritSampleTime=off
      settings: RTWStateStorageClass=Auto
  Memory1 : Memory  X0=0  InheritSampleTime=off
      settings: RTWStateStorageClass=Auto
  MinMax : MinMax  Function=min  Inputs=2
  TR Look-Up Table TR=Tout/Tin : Lookup  InputValues=htc_sr  OutputValues=htc_tr
  T_max : Subsystem
      settings: RTWFcnNameOpts=Auto  RTWFileNameOpts=Auto
  Tin*TR= Tout,req : Product  Inputs=2  Multiplication=Element-wise(.*)  SaturateOnIntegerOverflow=on
  engine speed estimator : Subsystem
      settings: RTWFcnNameOpts=Auto  RTWFileNameOpts=Auto
  "shifting, override zero Trequest" : Switch  Threshold=eps
  T req : Outport  Port=1
  wires:
  Tin*TR= Tout,req/1 -> Memory/1
  TR/1 -> Tin*TR= Tout,req/2
  Req'd  input trq/1 -> Tin*TR= Tout,req/1
  Memory/1 -> "shifting, override zero Trequest"/1
  T_max/1(T_max max gain from htc) -> MinMax/2
  "shifting, override zero Trequest"/1 -> MinMax/1
  TR Look-Up Table TR=Tout/Tin/1 -> T_max/2(TR)
  MinMax/1 -> T req/1
  engine speed estimator/1(Out1) -> T_max/1(w_APU)
  Memory1/1 -> TR Look-Up Table TR=Tout/Tin/1
  SR/1 -> Memory1/1
  htc_spd_in_a/1 -> engine speed estimator/1(htc_spd_in_a)
  Req'd output trq/1 -> "shifting, override zero Trequest"/3
  [shifting] -> "shifting, override zero Trequest"/2

== system lib_transmission2/hydraulic torque converter <htc> HEV/HTC for parallel HEV and Interface/model for parallel HEV/TR ==
  SR : Inport  Port=1  LatchInput=off
  coasting : Inport  Port=2  LatchInput=off
  1/SR*TR  for coast : Fcn  Expr=1/u
  Constant3 : Constant  Value=1
  Logical Operator : Logic  Operator=NOT  Inputs=1
  Logical Operator1 : Logic  Operator=NOT  Inputs=1
  TR Look-Up Table TR=Tout/Tin : Lookup  InputValues=htc_sr  OutputValues=htc_tr
  TR Look-Up Table TR=Tout/Tin coast : Lookup  InputValues=htc_sr_coast  OutputValues=htc_tr_coast
  To Workspace11 : ToWorkspace  VariableName=htc_efficiency  SampleTime=-1  SaveFormat=Array
  effic=SR*TR : Product  Inputs=**  Multiplication=Element-wise(.*)  SaturateOnIntegerOverflow=on
  if coasting : Switch  Threshold=eps
  if coasting1 : Switch  Threshold=eps
  "locked up, then TR=1" : Switch  Threshold=eps
  min,max : Saturate  UpperLimit=htc_max_coast_tr  LowerLimit=htc_min_coast_tr  LinearizeAsGain=on
  TR : Outport  Port=1  InitialOutput=0
  wires:
  if coasting1/1 -> To Workspace11/1
  1/SR*TR  for coast/1 -> if coasting1/3
  effic=SR*TR/1 -> 1/SR*TR  for coast/1, if coasting1/1
  Logical Operator1/1 -> if coasting1/2, if coasting/2
  if coasting/1 -> effic=SR*TR/2, TR/1
  coasting/1 -> Logical Operator1/1
  SR/1 -> effic=SR*TR/1, TR Look-Up Table TR=Tout/Tin/1, TR Look-Up Table TR=Tout/Tin coast/1
  min,max/1 -> if coasting/3
  TR Look-Up Table TR=Tout/Tin coast/1 -> min,max/1
  "locked up, then TR=1"/1 -> if coasting/1
  Logical Operator/1 -> "locked up, then TR=1"/2
  [locked_up] -> Logical Operator/1
  Constant3/1 -> "locked up, then TR=1"/3
  TR Look-Up Table TR=Tout/Tin/1 -> "locked up, then TR=1"/1

== system lib_transmission2/hydraulic torque converter <htc> HEV/HTC for parallel HEV and Interface/model for parallel HEV/effect of inertia (Nm) ==
  note: This block computes the torque required to overcome the inertia of the
      | turbine (plus 1/2 fluid in htc).
  turbine/output speed (rad/s) : Inport  Port=1  LatchInput=off
  Constant : Constant  Value=htc_inertia
  Product : Product  Inputs=2  Multiplication=Element-wise(.*)  SaturateOnIntegerOverflow=on
  d/dt : Derivative
  inertia torque (Nm) : Outport  Port=1  InitialOutput=0
  wires:
  Product/1 -> inertia torque (Nm)/1
  Constant/1 -> Product/2
  turbine/output speed (rad/s)/1 -> d/dt/1
  d/dt/1 -> Product/1

== system lib_transmission2/hydraulic torque converter <htc> HEV/HTC for parallel HEV and Interface/model for parallel HEV/enhancedToWorkspace ==
  In1 : Inport  Port=1  LatchInput=off
  Terminator : Terminator
  wires:
  In1/1 -> Terminator/1

== system lib_transmission2/hydraulic torque converter <htc> HEV/HTC for parallel HEV and Interface/model for parallel HEV/enhancedToWorkspace1 ==
  In1 : Inport  Port=1  LatchInput=off
  Terminator : Terminator
  wires:
  In1/1 -> Terminator/1

== system lib_transmission2/hydraulic torque converter <htc> HEV/HTC for parallel HEV and Interface/model for parallel HEV/enhancedToWorkspace10 ==
  In1 : Inport  Port=1  LatchInput=off
  Terminator : Terminator
  wires:
  In1/1 -> Terminator/1

== system lib_transmission2/hydraulic torque converter <htc> HEV/HTC for parallel HEV and Interface/model for parallel HEV/enhancedToWorkspace2 ==
  In1 : Inport  Port=1  LatchInput=off
  Terminator : Terminator
  wires:
  In1/1 -> Terminator/1

== system lib_transmission2/hydraulic torque converter <htc> HEV/HTC for parallel HEV and Interface/model for parallel HEV/enhancedToWorkspace3 ==
  In1 : Inport  Port=1  LatchInput=off
  Terminator : Terminator
  wires:
  In1/1 -> Terminator/1

== system lib_transmission2/hydraulic torque converter <htc> HEV/HTC for parallel HEV and Interface/model for parallel HEV/enhancedToWorkspace4 ==
  In1 : Inport  Port=1  LatchInput=off
  Terminator : Terminator
  wires:
  In1/1 -> Terminator/1

== system lib_transmission2/hydraulic torque converter <htc> HEV/HTC for parallel HEV and Interface/model for parallel HEV/enhancedToWorkspace5 ==
  In1 : Inport  Port=1  LatchInput=off
  Terminator : Terminator
  wires:
  In1/1 -> Terminator/1

== system lib_transmission2/hydraulic torque converter <htc> HEV/HTC for parallel HEV and Interface/model for parallel HEV/enhancedToWorkspace6 ==
  In1 : Inport  Port=1  LatchInput=off
  Terminator : Terminator
  wires:
  In1/1 -> Terminator/1

== system lib_transmission2/hydraulic torque converter <htc> HEV/HTC for parallel HEV and Interface/model for parallel HEV/enhancedToWorkspace7 ==
  In1 : Inport  Port=1  LatchInput=off
  Terminator : Terminator
  wires:
  In1/1 -> Terminator/1

== system lib_transmission2/hydraulic torque converter <htc> HEV/HTC for parallel HEV and Interface/model for parallel HEV/enhancedToWorkspace8 ==
  In1 : Inport  Port=1  LatchInput=off
  Terminator : Terminator
  wires:
  In1/1 -> Terminator/1

== system lib_transmission2/hydraulic torque converter <htc> HEV/HTC for parallel HEV and Interface/model for parallel HEV/enhancedToWorkspace9 ==
  In1 : Inport  Port=1  LatchInput=off
  Terminator : Terminator
  wires:
  In1/1 -> Terminator/1

== system lib_transmission2/hydraulic torque converter <htc> with pump loss/conventional HTC  and Interface/htc model/Block NOTES ==
  note: This block predicts the relative speed of the HTC input (pump) and output
      | (turbine).  Torque converter lockup is modeled.
      |
      | 1/24/00:tm updated gear_ratio flag to shifting flag
      |
      | 02/19/03: zz added pump loss
